simulink model "VehicleSteering_sim_ObserverDesign"  (R2020a)
settings: Solver=VariableStepAuto  StartTime=0.0  StopTime=10.0  RelTol=1e-3
InitFcn:
  | VehicleSteering_ObserverDesign
undefined symbols (not defined in the file): A, B, C, D, K, kr, L
settings Model: Creator=jofr  LastModifiedBy=rizwanahmed
settings DataIOCC: ReturnWorkspaceOutputs=off
settings DebuggingCC: ArithmeticOperatorsInVariantConditions=warning
settings SFSimCC: SimUseLocalCustomCode=off  CustomCodeUndefinedFunction=UseInterfaceOnly
settings RTWCC: RTWUseLocalCustomCode=off

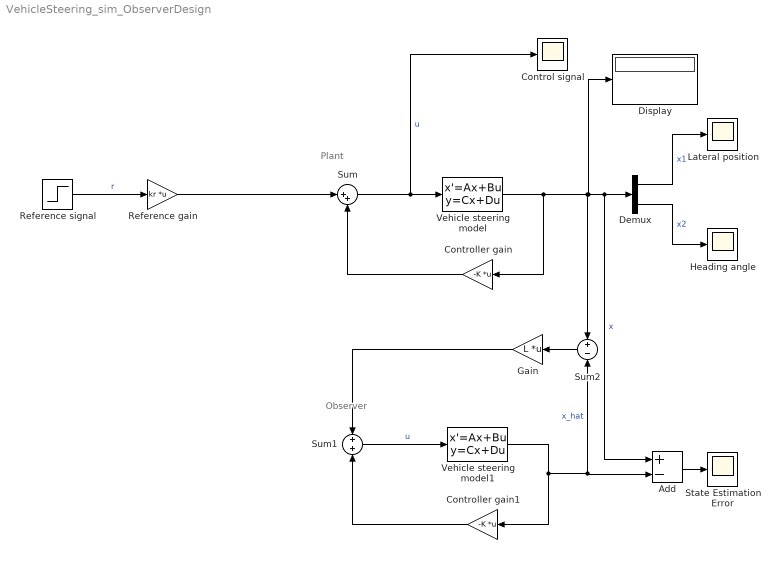
== system VehicleSteering_sim_ObserverDesign ==
  note: Plant
  note: Observer
  Add : Sum  Inputs=+-
  Control signal : Scope
  Controller gain : Gain  Gain=-K  Multiplication=Matrix(K*u)
  Controller gain1 : Gain  Gain=-K  Multiplication=Matrix(K*u)
  Demux : Demux  Outputs=2
  Display : Display
  Gain : Gain  Gain=L  Multiplication=Matrix(K*u)
  Heading angle : Scope
  Lateral position : Scope
  Reference gain : Gain  Gain=kr  Multiplication=Matrix(K*u)
  "Reference signal " : Step  SampleTime=0
  State Estimation Error : Scope
  Sum : Sum  Inputs=|++
  Sum1 : Sum
  Sum2 : Sum  Inputs=+-
  Vehicle steering model : StateSpace  A=A  B=B  C=C  D=D  InitialCondition=0
  Vehicle steering model1 : StateSpace  A=A  B=B  C=C  D=D  InitialCondition=0
  wires:
  Vehicle steering model/1 -> Display/1, Add/1, Demux/1, Sum2/1, Controller gain/1  "x"
  Sum/1 -> Control signal/1, Vehicle steering model/1  "u"
  Controller gain/1 -> Sum/2
  Demux/1 -> Lateral position/1  "x1"
  Demux/2 -> Heading angle/1  "x2"
  "Reference signal "/1 -> Reference gain/1  "r"
  Sum1/1 -> Vehicle steering model1/1  "u"
  Reference gain/1 -> Sum/1
  Vehicle steering model1/1 -> Controller gain1/1, Add/2, Sum2/2  "x_hat"
  Sum2/1 -> Gain/1
  Gain/1 -> Sum1/1
  Controller gain1/1 -> Sum1/2
  Add/1 -> State Estimation Error/1
